simulink model "simulacion_motor"  (Simulink 7.0)
settings: Solver=ode45  StartTime=0.0  StopTime=5  RelTol=1e-3
values from neighbouring files (symbols this model uses):
  Ts = 0.001    [Ejercicio2.m]
settings Model: Creator=alumno  LastModifiedBy=alumno

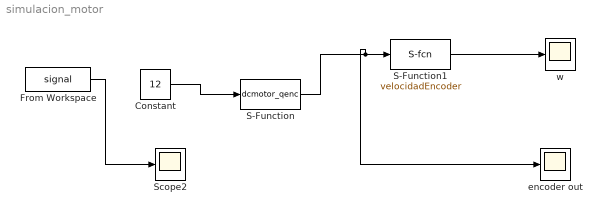
== system simulacion_motor ==
  Constant : Constant  Value=12  OutDataType=sfix(16)  OutScaling=2^0
  From Workspace : FromWorkspace  VariableName=signal  SampleTime=Ts
  S-Function : S-Function  FunctionName=dcmotor_qenc  Parameters=1
  S-Function1 : S-Function  FunctionName=velocidadEncoder  Parameters=1
  Scope2 : Scope
      settings: SaveName=ScopeData2
  encoder out : Scope
  w : Scope
  wires:
  S-Function/1 -> S-Function1/1, encoder out/1
  Constant/1 -> S-Function/1
  From Workspace/1 -> Scope2/1
  S-Function1/1 -> w/1
